simulink model "Dron_pid_XY"  (R2019a)
settings: Solver=FixedStepAuto  StartTime=0.0  StopTime=100  FixedStep=1e-5  RelTol=1e-3
values from neighbouring files (symbols this model uses):
  b = force_max_1 / omega_max ^ 2    (= 6.86183516529e-08)    [dron.m]
  d = 2e-9    (= 2e-09)    [dron.m]
  delay = 0.001    [dron.m]
  force_max = force_max_1 * 4    (= 47.088)    [dron.m]
  g = 9.81    [dron.m]
  Ixx = 0.02276    [dron.m]
  Iyy = Ixx    (= 0.02276)    [dron.m]
  Izz = 0.03132    [dron.m]
  k_x = 10    [dron.m]
  k_y = 10    [dron.m]
  k_z = 1    [dron.m]
  l = 0.225    [dron.m]
  m = 1    [dron.m]
  omega_max = 13098    [dron.m]
  torque_max_rp = omega_max ^ 2 * 2 * b * l    (= 5.2974)    [dron.m]
  torque_max_y = omega_max ^ 2 * 2 * d    (= 0.686230416)    [dron.m]
undefined symbols (not defined in the file or in its folder): sigbuilder_block
libraries: simulink_extras x9, simulink x6, powerlib_extras x1
settings Model: Creator=alber  LastModifiedBy=alber
settings DataIOCC: ReturnWorkspaceOutputs=off

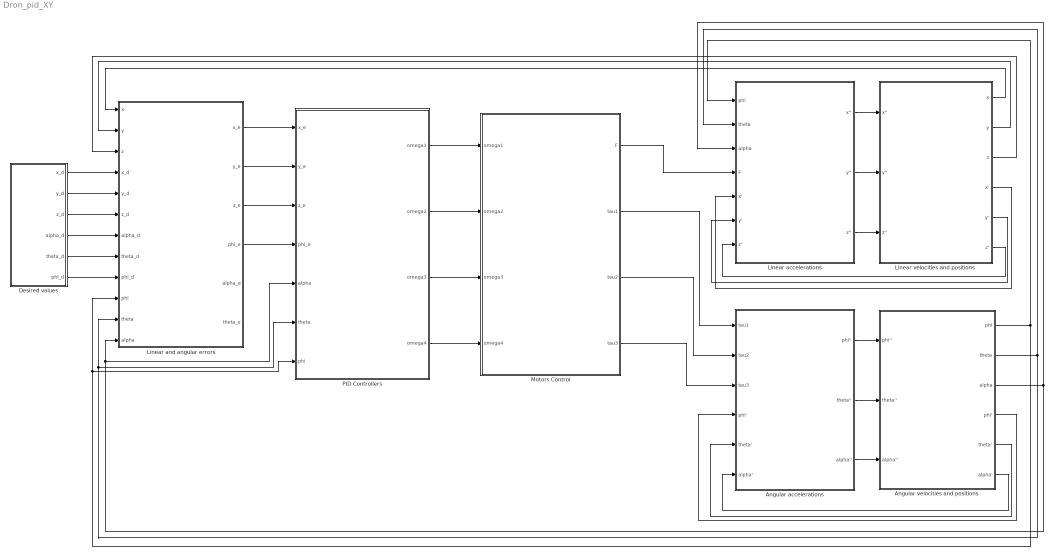
== system Dron_pid_XY ==
  Angular accelerations : Subsystem
  Angular velocities and positions : Subsystem
  Desired values : Subsystem
  Linear accelerations : Subsystem
  Linear and angular errors : Subsystem
  Linear velocities and positions : Subsystem
  Motors Control : Subsystem
  PID Controllers : Subsystem
  wires:
  Angular accelerations/1(phi'') -> Angular velocities and positions/1(phi'')
  Angular accelerations/2(theta'') -> Angular velocities and positions/2(theta'')
  Angular accelerations/3(alpha'') -> Angular velocities and positions/3(alpha'')
  Desired values/4(alpha_d) -> Linear and angular errors/7(alpha_d)
  Desired values/5(theta_d) -> Linear and angular errors/8(theta_d)
  Desired values/6(phi_d) -> Linear and angular errors/9(phi_d)
  Linear accelerations/3(z'') -> Linear velocities and positions/3(z'')
  Linear accelerations/2(y'') -> Linear velocities and positions/2(y'')
  Linear accelerations/1(x'') -> Linear velocities and positions/1(x'')
  Linear and angular errors/1(x_e) -> PID Controllers/1(x_e)
  Linear and angular errors/2(y_e) -> PID Controllers/2(y_e)
  Linear and angular errors/3(z_e) -> PID Controllers/3(z_e)
  Linear and angular errors/4(phi_e) -> PID Controllers/4(phi_e)
  PID Controllers/1(omega1) -> Motors Control/1(omega1)
  PID Controllers/2(omega2) -> Motors Control/2(omega2)
  PID Controllers/3(omega3) -> Motors Control/3(omega3)
  PID Controllers/4(omega4) -> Motors Control/4(omega4)
  Linear velocities and positions/6(z') -> Linear accelerations/7(z')
  Linear velocities and positions/5(y') -> Linear accelerations/6(y')
  Linear velocities and positions/4(x') -> Linear accelerations/5(x')
  Linear velocities and positions/1(x) -> Linear and angular errors/1(x)
  Linear velocities and positions/2(y) -> Linear and angular errors/2(y)
  Linear velocities and positions/3(z) -> Linear and angular errors/3(z)
  Angular velocities and positions/6(alpha') -> Angular accelerations/6(alpha')
  Angular velocities and positions/5(theta') -> Angular accelerations/5(theta')
  Angular velocities and positions/4(phi') -> Angular accelerations/4(phi')
  Motors Control/2(tau1) -> Angular accelerations/1(tau1)
  Motors Control/3(tau2) -> Angular accelerations/2(tau2)
  Motors Control/4(tau3) -> Angular accelerations/3(tau3)
  Motors Control/1(F) -> Linear accelerations/4(F)
  Angular velocities and positions/3(alpha) -> Linear accelerations/3(alpha), PID Controllers/5(alpha), Linear and angular errors/12(alpha)
  Angular velocities and positions/2(theta) -> Linear accelerations/2(theta), PID Controllers/6(theta), Linear and angular errors/11(theta)
  Angular velocities and positions/1(phi) -> Linear accelerations/1(phi), PID Controllers/7(phi), Linear and angular errors/10(phi)
  Desired values/1(x_d) -> Linear and angular errors/4(x_d)
  Desired values/2(y_d) -> Linear and angular errors/5(y_d)
  Desired values/3(z_d) -> Linear and angular errors/6(z_d)

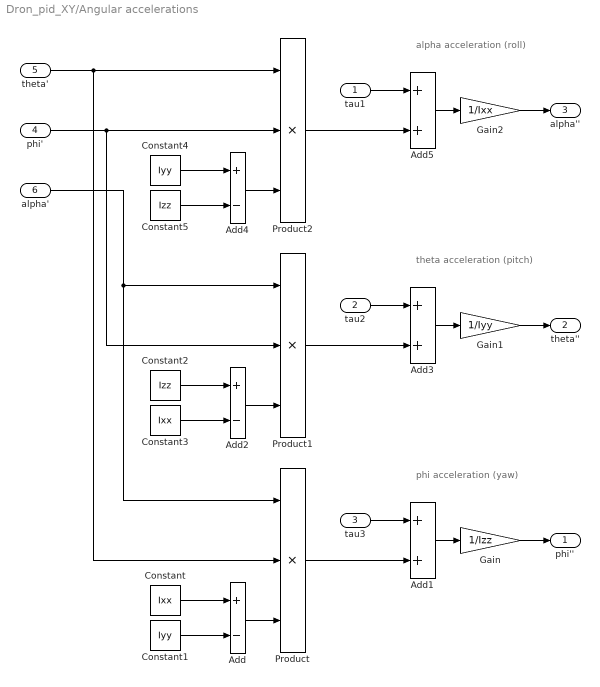
== system Dron_pid_XY/Angular accelerations ==
  note: alpha acceleration (roll)
  note: theta acceleration (pitch)
  note: phi acceleration (yaw)
  tau1 : Inport
  tau2 : Inport  Port=2
  tau3 : Inport  Port=3
  phi' : Inport  Port=4
  theta' : Inport  Port=5
  alpha' : Inport  Port=6
  Add : Sum  Inputs=+-
  Add1 : Sum
  Add2 : Sum  Inputs=+-
  Add3 : Sum
  Add4 : Sum  Inputs=+-
  Add5 : Sum
  Constant : Constant  Value=Ixx
  Constant1 : Constant  Value=Iyy
  Constant2 : Constant  Value=Izz
  Constant3 : Constant  Value=Ixx
  Constant4 : Constant  Value=Iyy
  Constant5 : Constant  Value=Izz
  Gain : Gain  Gain=1/Izz
  Gain1 : Gain  Gain=1/Iyy
  Gain2 : Gain  Gain=1/Ixx
  Product : Product  Inputs=3
  Product1 : Product  Inputs=3
  Product2 : Product  Inputs=3
  phi'' : Outport
  theta'' : Outport  Port=2
  alpha'' : Outport  Port=3
  wires:
  Constant2/1 -> Add2/1
  Add3/1 -> Gain1/1
  Constant1/1 -> Add/2
  Product2/1 -> Add5/2
  tau1/1 -> Add5/1
  Add1/1 -> Gain/1
  Add/1 -> Product/3
  Constant/1 -> Add/1
  Constant5/1 -> Add4/2
  Product1/1 -> Add3/2
  Add2/1 -> Product1/3
  tau2/1 -> Add3/1
  Constant3/1 -> Add2/2
  Add5/1 -> Gain2/1
  tau3/1 -> Add1/1
  Product/1 -> Add1/2
  Constant4/1 -> Add4/1
  Add4/1 -> Product2/3
  Gain2/1 -> alpha''/1
  Gain1/1 -> theta''/1
  Gain/1 -> phi''/1
  theta'/1 -> Product/2, Product2/1
  phi'/1 -> Product1/2, Product2/2
  alpha'/1 -> Product/1, Product1/1

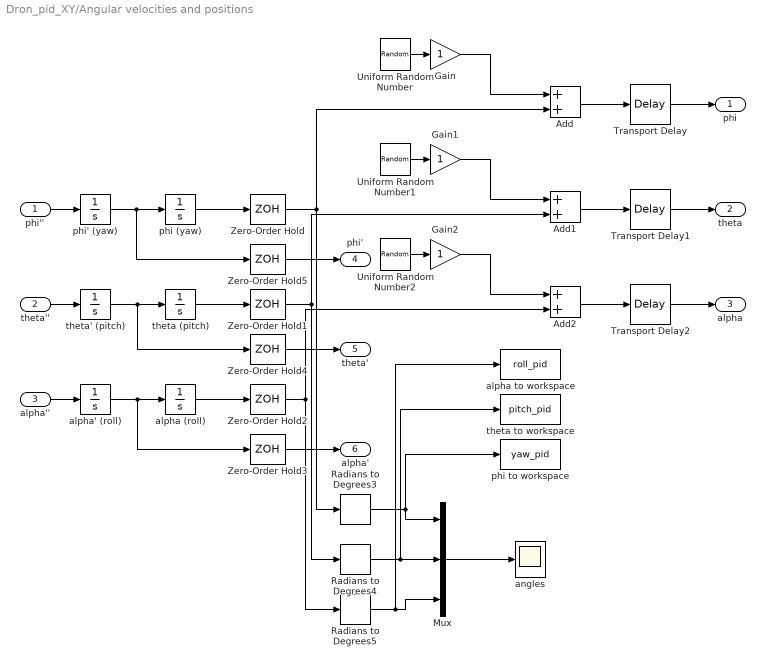
== system Dron_pid_XY/Angular velocities and positions ==
  phi'' : Inport
  theta'' : Inport  Port=2
  alpha'' : Inport  Port=3
  Add : Sum
  Add1 : Sum
  Add2 : Sum
  Gain : Gain
  Gain1 : Gain
  Gain2 : Gain
  Mux : Mux  Inputs=3
  Radians to Degrees3 : simulink_extras/Transformations/Radians to Degrees
  Radians to Degrees4 : simulink_extras/Transformations/Radians to Degrees
  Radians to Degrees5 : simulink_extras/Transformations/Radians to Degrees
  Transport Delay : TransportDelay  DelayTime=delay
  Transport Delay1 : TransportDelay  DelayTime=delay
  Transport Delay2 : TransportDelay  DelayTime=delay
  Uniform Random Number : UniformRandomNumber  Minimum=-0.005  Maximum=0.005  SampleTime=1e-4
  Uniform Random Number1 : UniformRandomNumber  Minimum=-0.005  Maximum=0.005  SampleTime=1e-4
  Uniform Random Number2 : UniformRandomNumber  Minimum=-0.005  Maximum=0.005  SampleTime=1e-4
  Zero-Order Hold{,1..5} (6 alike) : ZeroOrderHold  SampleTime=1e-4
  alpha (roll) : Integrator  LimitOutput=on  UpperSaturationLimit=pi  LowerSaturationLimit=-pi
  alpha to workspace : ToWorkspace  VariableName=roll_pid  SampleTime=1e-5
  alpha' (roll) : Integrator
  angles : Scope
  phi (yaw) : Integrator  LimitOutput=on  UpperSaturationLimit=pi  LowerSaturationLimit=-pi
  phi to workspace : ToWorkspace  VariableName=yaw_pid  SampleTime=1e-5
  phi' (yaw) : Integrator
  "theta (pitch) " : Integrator  LimitOutput=on  UpperSaturationLimit=pi  LowerSaturationLimit=-pi
  theta to workspace : ToWorkspace  VariableName=pitch_pid  SampleTime=1e-5
  theta' (pitch) : Integrator
  phi : Outport
  theta : Outport  Port=2
  alpha : Outport  Port=3
  phi' : Outport  Port=4
  theta' : Outport  Port=5
  alpha' : Outport  Port=6
  wires:
  phi (yaw)/1 -> Zero-Order Hold/1
  alpha' (roll)/1 -> Zero-Order Hold3/1, alpha (roll)/1
  theta' (pitch)/1 -> Zero-Order Hold4/1, "theta (pitch) "/1
  "theta (pitch) "/1 -> Zero-Order Hold1/1
  phi' (yaw)/1 -> Zero-Order Hold5/1, phi (yaw)/1
  theta''/1 -> theta' (pitch)/1
  alpha''/1 -> alpha' (roll)/1
  Zero-Order Hold1/1 -> Add1/2, Radians to Degrees4/1
  phi''/1 -> phi' (yaw)/1
  Zero-Order Hold/1 -> Radians to Degrees3/1, Add/2
  Zero-Order Hold2/1 -> Radians to Degrees5/1, Add2/2
  Radians to Degrees4/1 -> theta to workspace/1, Mux/2
  Radians to Degrees3/1 -> phi to workspace/1, Mux/1
  Radians to Degrees5/1 -> alpha to workspace/1, Mux/3
  Mux/1 -> angles/1
  alpha (roll)/1 -> Zero-Order Hold2/1
  Zero-Order Hold3/1 -> alpha'/1
  Zero-Order Hold4/1 -> theta'/1
  Zero-Order Hold5/1 -> phi'/1
  Uniform Random Number/1 -> Gain/1
  Uniform Random Number1/1 -> Gain1/1
  Uniform Random Number2/1 -> Gain2/1
  Add/1 -> Transport Delay/1
  Add1/1 -> Transport Delay1/1
  Add2/1 -> Transport Delay2/1
  Gain/1 -> Add/1
  Gain1/1 -> Add1/1
  Gain2/1 -> Add2/1
  Transport Delay/1 -> phi/1
  Transport Delay1/1 -> theta/1
  Transport Delay2/1 -> alpha/1

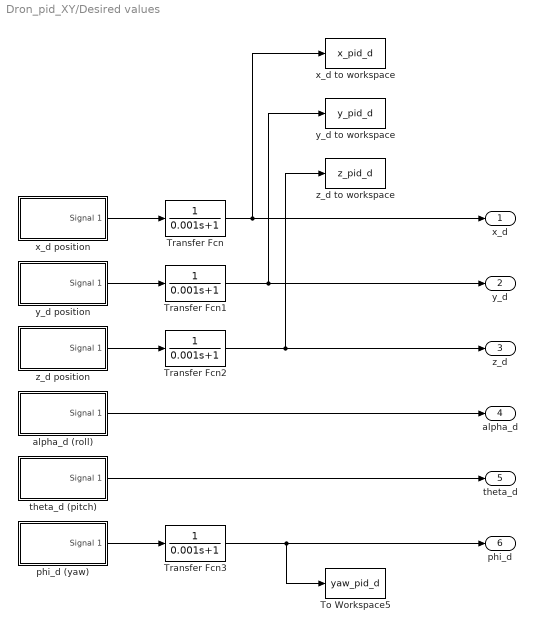
== system Dron_pid_XY/Desired values ==
  To Workspace5 : ToWorkspace  VariableName=yaw_pid_d  SampleTime=1e-5
  Transfer Fcn{,1..3} (4 alike) : TransferFcn  Denominator=[0.001 1]
  alpha_d (roll) : Subsystem  Tag=STV Subsys  LoadFcn=sigbuilder_block('load');  StartFcn=sigbuilder_block('start');  StopFcn=sigbuilder_block('stop');  ClipboardFcn=sigbuilder_block('clipboard');  mask(Sigbuilder block){tuvar=[0:10]}
      mask help: Simulink:masks:SigbuilderBlock_MD
      mask init:
      | if ~strcmp(get_param(bdroot(gcbh),'SimulationStatus'),'stopped') tuvar = sigbuilder_block('maskInit'); end
      settings: CopyFcn=sigbuilder_block('copy');  DeleteFcn=sigbuilder_block('delete');  ModelCloseFcn=sigbuilder_block('modelClose');  PreSaveFcn=sigbuilder_block('preSave');  PauseFcn=sigbuilder_block('pause');  ContinueFcn=sigbuilder_block('continue');  NameChangeFcn=sigbuilder_block('namechange');  OpenFcn=sigbuilder_block('open',[150.6 124.8 550.8 400.2 ]);  CloseFcn=sigbuilder_block('close');
      mask Display: plot(0, 0, 100, 100,[2, 2, 32, 32, 2], [68, 8, 8, 68, 68],[32, 2], [38, 38], [32, 19, 2],[53, 60, 44], [32, 17, 17, 2],[16, 16, 31, 31]);txt = getActiveGroup(gcbh);text(2, 100, txt,'verticalAlignment', 'top');
  phi_d (yaw) : Subsystem  Tag=STV Subsys  LoadFcn=sigbuilder_block('load');  StartFcn=sigbuilder_block('start');  StopFcn=sigbuilder_block('stop');  ClipboardFcn=sigbuilder_block('clipboard');  mask(Sigbuilder block){tuvar=[0:10]}
      mask help: Simulink:masks:SigbuilderBlock_MD
      mask init:
      | if ~strcmp(get_param(bdroot(gcbh),'SimulationStatus'),'stopped') tuvar = sigbuilder_block('maskInit'); end
      settings: CopyFcn=sigbuilder_block('copy');  DeleteFcn=sigbuilder_block('delete');  ModelCloseFcn=sigbuilder_block('modelClose');  PreSaveFcn=sigbuilder_block('preSave');  PauseFcn=sigbuilder_block('pause');  ContinueFcn=sigbuilder_block('continue');  NameChangeFcn=sigbuilder_block('namechange');  OpenFcn=sigbuilder_block('open',[595.8 77.4 550.8 361.2 ]);  CloseFcn=sigbuilder_block('close');
      mask Display: plot(0, 0, 100, 100,[2, 2, 32, 32, 2], [68, 8, 8, 68, 68],[32, 2], [38, 38], [32, 19, 2],[53, 60, 44], [32, 17, 17, 2],[16, 16, 31, 31]);txt = getActiveGroup(gcbh);text(2, 100, txt,'verticalAlignment', 'top');
  theta_d (pitch) : Subsystem  Tag=STV Subsys  LoadFcn=sigbuilder_block('load');  StartFcn=sigbuilder_block('start');  StopFcn=sigbuilder_block('stop');  ClipboardFcn=sigbuilder_block('clipboard');  mask(Sigbuilder block){tuvar=[0:10]}
      mask help: Simulink:masks:SigbuilderBlock_MD
      mask init:
      | if ~strcmp(get_param(bdroot(gcbh),'SimulationStatus'),'stopped') tuvar = sigbuilder_block('maskInit'); end
      settings: CopyFcn=sigbuilder_block('copy');  DeleteFcn=sigbuilder_block('delete');  ModelCloseFcn=sigbuilder_block('modelClose');  PreSaveFcn=sigbuilder_block('preSave');  PauseFcn=sigbuilder_block('pause');  ContinueFcn=sigbuilder_block('continue');  NameChangeFcn=sigbuilder_block('namechange');  OpenFcn=sigbuilder_block('open',[583.2 81.6 550.8 400.2 ]);  CloseFcn=sigbuilder_block('close');
      mask Display: plot(0, 0, 100, 100,[2, 2, 32, 32, 2], [68, 8, 8, 68, 68],[32, 2], [38, 38], [32, 19, 2],[53, 60, 44], [32, 17, 17, 2],[16, 16, 31, 31]);txt = getActiveGroup(gcbh);text(2, 100, txt,'verticalAlignment', 'top');
  x_d position : Subsystem  Tag=STV Subsys  LoadFcn=sigbuilder_block('load');  StartFcn=sigbuilder_block('start');  StopFcn=sigbuilder_block('stop');  ClipboardFcn=sigbuilder_block('clipboard');  mask(Sigbuilder block){tuvar=[0:10]}
      mask help: Simulink:masks:SigbuilderBlock_MD
      mask init:
      | if ~strcmp(get_param(bdroot(gcbh),'SimulationStatus'),'stopped') tuvar = sigbuilder_block('maskInit'); end
      settings: CopyFcn=sigbuilder_block('copy');  DeleteFcn=sigbuilder_block('delete');  ModelCloseFcn=sigbuilder_block('modelClose');  PreSaveFcn=sigbuilder_block('preSave');  PauseFcn=sigbuilder_block('pause');  ContinueFcn=sigbuilder_block('continue');  NameChangeFcn=sigbuilder_block('namechange');  OpenFcn=sigbuilder_block('open',[0.75 0.75 718.5 745.5 ]);  CloseFcn=sigbuilder_block('close');
      mask Display: plot(0, 0, 100, 100,[2, 2, 32, 32, 2], [68, 8, 8, 68, 68],[32, 2], [38, 38], [32, 19, 2],[53, 60, 44], [32, 17, 17, 2],[16, 16, 31, 31]);txt = getActiveGroup(gcbh);text(2, 100, txt,'verticalAlignment', 'top');
  x_d to workspace : ToWorkspace  VariableName=x_pid_d  SampleTime=1e-5
  y_d position : Subsystem  Tag=STV Subsys  LoadFcn=sigbuilder_block('load');  StartFcn=sigbuilder_block('start');  StopFcn=sigbuilder_block('stop');  ClipboardFcn=sigbuilder_block('clipboard');  mask(Sigbuilder block){tuvar=[0:10]}
      mask help: Simulink:masks:SigbuilderBlock_MD
      mask init:
      | if ~strcmp(get_param(bdroot(gcbh),'SimulationStatus'),'stopped') tuvar = sigbuilder_block('maskInit'); end
      settings: CopyFcn=sigbuilder_block('copy');  DeleteFcn=sigbuilder_block('delete');  ModelCloseFcn=sigbuilder_block('modelClose');  PreSaveFcn=sigbuilder_block('preSave');  PauseFcn=sigbuilder_block('pause');  ContinueFcn=sigbuilder_block('continue');  NameChangeFcn=sigbuilder_block('namechange');  OpenFcn=sigbuilder_block('open',[0.75 0.75 718.5 745.5 ]);  CloseFcn=sigbuilder_block('close');
      mask Display: plot(0, 0, 100, 100,[2, 2, 32, 32, 2], [68, 8, 8, 68, 68],[32, 2], [38, 38], [32, 19, 2],[53, 60, 44], [32, 17, 17, 2],[16, 16, 31, 31]);txt = getActiveGroup(gcbh);text(2, 100, txt,'verticalAlignment', 'top');
  y_d to workspace : ToWorkspace  VariableName=y_pid_d  SampleTime=1e-5
  z_d position : Subsystem  Tag=STV Subsys  LoadFcn=sigbuilder_block('load');  StartFcn=sigbuilder_block('start');  StopFcn=sigbuilder_block('stop');  ClipboardFcn=sigbuilder_block('clipboard');  mask(Sigbuilder block){tuvar=[0:10]}
      mask help: Simulink:masks:SigbuilderBlock_MD
      mask init:
      | if ~strcmp(get_param(bdroot(gcbh),'SimulationStatus'),'stopped') tuvar = sigbuilder_block('maskInit'); end
      settings: CopyFcn=sigbuilder_block('copy');  DeleteFcn=sigbuilder_block('delete');  ModelCloseFcn=sigbuilder_block('modelClose');  PreSaveFcn=sigbuilder_block('preSave');  PauseFcn=sigbuilder_block('pause');  ContinueFcn=sigbuilder_block('continue');  NameChangeFcn=sigbuilder_block('namechange');  OpenFcn=sigbuilder_block('open',[112.5 10.5 574.5 585.75 ]);  CloseFcn=sigbuilder_block('close');
      mask Display: plot(0, 0, 100, 100,[2, 2, 32, 32, 2], [68, 8, 8, 68, 68],[32, 2], [38, 38], [32, 19, 2],[53, 60, 44], [32, 17, 17, 2],[16, 16, 31, 31]);txt = getActiveGroup(gcbh);text(2, 100, txt,'verticalAlignment', 'top');
  z_d to workspace : ToWorkspace  VariableName=z_pid_d  SampleTime=1e-5
  x_d : Outport
  y_d : Outport  Port=2
  z_d : Outport  Port=3
  alpha_d : Outport  Port=4
  theta_d : Outport  Port=5
  phi_d : Outport  Port=6
  wires:
  alpha_d (roll)/1(Signal 1) -> alpha_d/1
  phi_d (yaw)/1(Signal 1) -> Transfer Fcn3/1
  theta_d (pitch)/1(Signal 1) -> theta_d/1
  z_d position/1(Signal 1) -> Transfer Fcn2/1
  y_d position/1(Signal 1) -> Transfer Fcn1/1
  x_d position/1(Signal 1) -> Transfer Fcn/1
  Transfer Fcn/1 -> x_d/1, x_d to workspace/1
  Transfer Fcn1/1 -> y_d/1, y_d to workspace/1
  Transfer Fcn2/1 -> z_d/1, z_d to workspace/1
  Transfer Fcn3/1 -> phi_d/1, To Workspace5/1

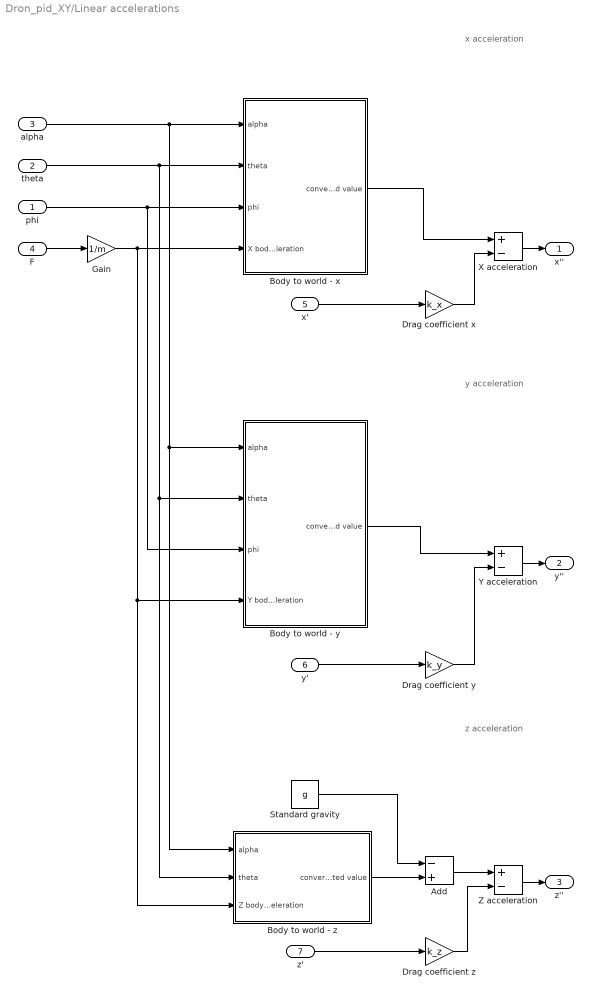
== system Dron_pid_XY/Linear accelerations ==
  note: z acceleration
  note: y acceleration
  note: x acceleration
  phi : Inport
  theta : Inport  Port=2
  alpha : Inport  Port=3
  F : Inport  Port=4
  x' : Inport  Port=5
  y' : Inport  Port=6
  z' : Inport  Port=7
  Add : Sum  Inputs=-+
  Body to world - x : Subsystem
  Body to world - y : Subsystem
  Body to world - z : Subsystem
  Drag coefficient x : Gain  Gain=k_x
  Drag coefficient y : Gain  Gain=k_y
  Drag coefficient z : Gain  Gain=k_z
  Gain : Gain  Gain=1/m
  Standard gravity : Constant  Value=g
  X acceleration : Sum  Inputs=+-
  Y acceleration : Sum  Inputs=+-
  Z acceleration : Sum  Inputs=+-
  x'' : Outport
  y'' : Outport  Port=2
  z'' : Outport  Port=3
  wires:
  theta/1 -> Body to world - z/2(theta), Body to world - y/2(theta), Body to world - x/2(theta)
  alpha/1 -> Body to world - z/1(alpha), Body to world - y/1(alpha), Body to world - x/1(alpha)
  phi/1 -> Body to world - y/3(phi), Body to world - x/3("phi ")
  Body to world - z/1(converted value) -> Add/2
  Standard gravity/1 -> Add/1
  F/1 -> Gain/1
  Add/1 -> Z acceleration/1
  Z acceleration/1 -> z''/1
  Y acceleration/1 -> y''/1
  X acceleration/1 -> x''/1
  Drag coefficient z/1 -> Z acceleration/2
  Drag coefficient y/1 -> Y acceleration/2
  Drag coefficient x/1 -> X acceleration/2
  Gain/1 -> Body to world - z/3(Z body acceleration), Body to world - y/4(Y body acceleration), Body to world - x/4(X body acceleration)
  Body to world - x/1(converted value) -> X acceleration/1
  Body to world - y/1(converted value) -> Y acceleration/1
  x'/1 -> Drag coefficient x/1
  y'/1 -> Drag coefficient y/1
  z'/1 -> Drag coefficient z/1

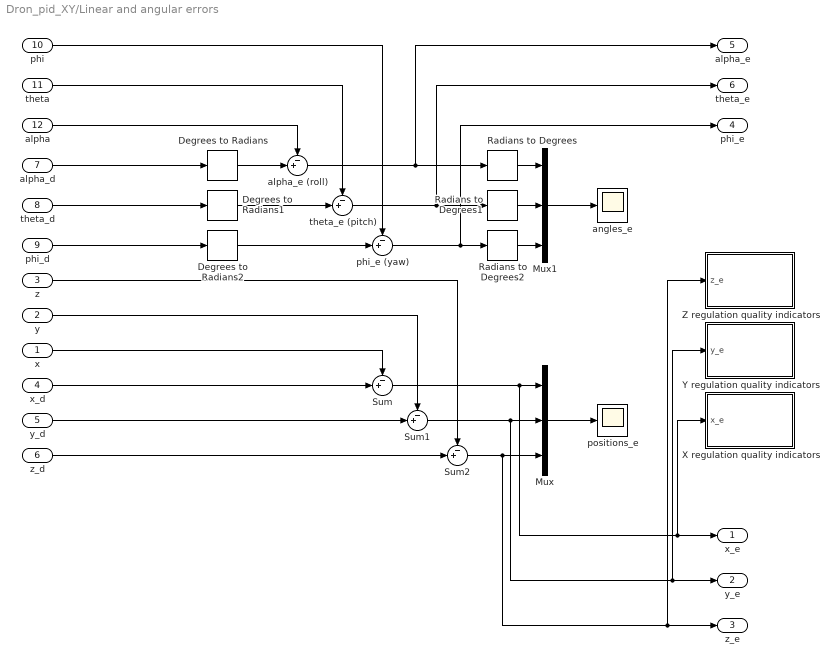
== system Dron_pid_XY/Linear and angular errors ==
  x : Inport
  y : Inport  Port=2
  z : Inport  Port=3
  x_d : Inport  Port=4
  y_d : Inport  Port=5
  z_d : Inport  Port=6
  alpha_d : Inport  Port=7
  theta_d : Inport  Port=8
  phi_d : Inport  Port=9
  phi : Inport  Port=10
  theta : Inport  Port=11
  alpha : Inport  Port=12
  Degrees to Radians : simulink_extras/Transformations/Degrees to Radians
  Degrees to Radians1 : simulink_extras/Transformations/Degrees to Radians
  Degrees to Radians2 : simulink_extras/Transformations/Degrees to Radians
  Mux : Mux  Inputs=3
  Mux1 : Mux  Inputs=3
  Radians to Degrees : simulink_extras/Transformations/Radians to Degrees
  Radians to Degrees1 : simulink_extras/Transformations/Radians to Degrees
  Radians to Degrees2 : simulink_extras/Transformations/Radians to Degrees
  Sum : Sum  Inputs=-+|
  Sum1 : Sum  Inputs=-+|
  Sum2 : Sum  Inputs=-+|
  X regulation quality indicators : Subsystem
  Y regulation quality indicators : Subsystem
  Z regulation quality indicators : Subsystem
  alpha_e (roll) : Sum  Inputs=-+|
  angles_e : Scope
  phi_e (yaw) : Sum  Inputs=-+|
  positions_e : Scope
  theta_e (pitch) : Sum  Inputs=-+|
  x_e : Outport
  y_e : Outport  Port=2
  z_e : Outport  Port=3
  phi_e : Outport  Port=4
  alpha_e : Outport  Port=5
  theta_e : Outport  Port=6
  wires:
  Mux1/1 -> angles_e/1
  Radians to Degrees/1 -> Mux1/1
  Radians to Degrees1/1 -> Mux1/2
  Radians to Degrees2/1 -> Mux1/3
  Sum/1 -> X regulation quality indicators/1(x_e), x_e/1, Mux/1
  Sum1/1 -> Y regulation quality indicators/1(y_e), y_e/1, Mux/2
  alpha_e (roll)/1 -> alpha_e/1, Radians to Degrees/1
  theta_e (pitch)/1 -> theta_e/1, Radians to Degrees1/1
  phi_e (yaw)/1 -> phi_e/1, Radians to Degrees2/1
  alpha_d/1 -> Degrees to Radians/1
  theta_d/1 -> Degrees to Radians1/1
  phi_d/1 -> Degrees to Radians2/1
  z_d/1 -> Sum2/2
  y_d/1 -> Sum1/2
  alpha/1 -> alpha_e (roll)/1
  theta/1 -> theta_e (pitch)/1
  phi/1 -> phi_e (yaw)/1
  x/1 -> Sum/1
  y/1 -> Sum1/1
  z/1 -> Sum2/1
  Mux/1 -> positions_e/1
  Degrees to Radians/1 -> alpha_e (roll)/2
  Degrees to Radians1/1 -> theta_e (pitch)/2
  Degrees to Radians2/1 -> phi_e (yaw)/2
  x_d/1 -> Sum/2
  Sum2/1 -> Z regulation quality indicators/1(z_e), z_e/1, Mux/3

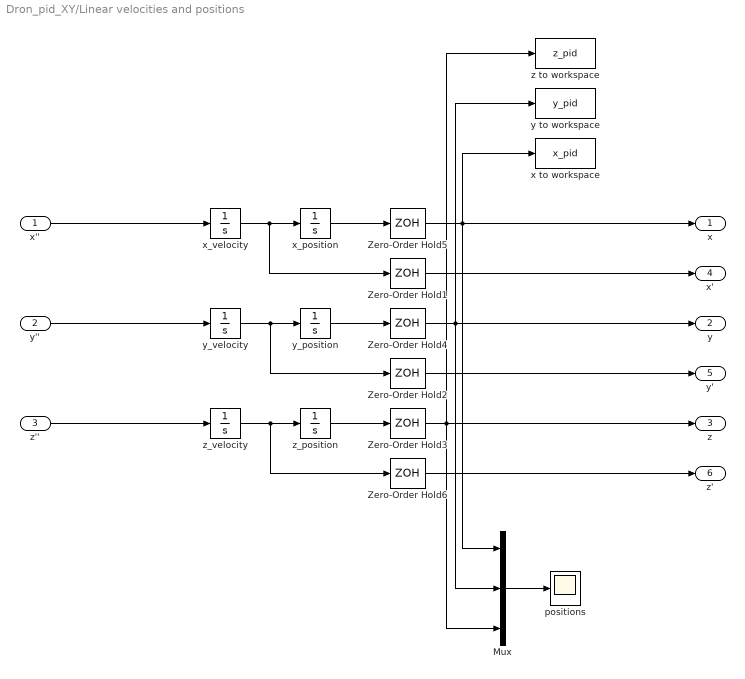
== system Dron_pid_XY/Linear velocities and positions ==
  x'' : Inport
  y'' : Inport  Port=2
  z'' : Inport  Port=3
  Mux : Mux  Inputs=3
  Zero-Order Hold{1..6} (6 alike) : ZeroOrderHold  SampleTime=1e-4
  positions : Scope
  x to workspace : ToWorkspace  VariableName=x_pid  SampleTime=1e-5
  x_position : Integrator
  x_velocity : Integrator
  y to workspace : ToWorkspace  VariableName=y_pid  SampleTime=1e-5
  y_position : Integrator
  y_velocity : Integrator
  z to workspace : ToWorkspace  VariableName=z_pid  SampleTime=1e-5
  z_position : Integrator  LimitOutput=on  LowerSaturationLimit=0
  z_velocity : Integrator
  x : Outport
  y : Outport  Port=2
  z : Outport  Port=3
  x' : Outport  Port=4
  y' : Outport  Port=5
  z' : Outport  Port=6
  wires:
  x_velocity/1 -> Zero-Order Hold1/1, x_position/1
  z_position/1 -> Zero-Order Hold3/1
  Zero-Order Hold4/1 -> Mux/2, y to workspace/1, y/1
  Zero-Order Hold5/1 -> x to workspace/1, Mux/1, x/1
  y_position/1 -> Zero-Order Hold4/1
  z_velocity/1 -> Zero-Order Hold6/1, z_position/1
  y_velocity/1 -> Zero-Order Hold2/1, y_position/1
  x_position/1 -> Zero-Order Hold5/1
  x''/1 -> x_velocity/1
  z''/1 -> z_velocity/1
  y''/1 -> y_velocity/1
  Zero-Order Hold3/1 -> Mux/3, z to workspace/1, z/1
  Mux/1 -> positions/1
  Zero-Order Hold1/1 -> x'/1
  Zero-Order Hold2/1 -> y'/1
  Zero-Order Hold6/1 -> z'/1

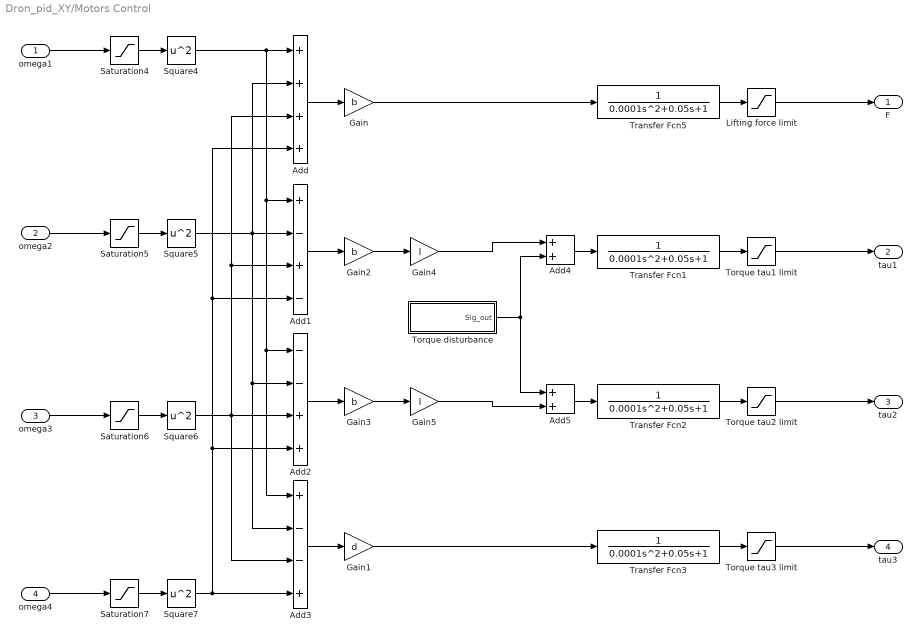
== system Dron_pid_XY/Motors Control ==
  omega1 : Inport
  omega2 : Inport  Port=2
  omega3 : Inport  Port=3
  omega4 : Inport  Port=4
  Add : Sum  Inputs=4
  Add1 : Sum  Inputs=+-+-
  Add2 : Sum  Inputs=--++
  Add3 : Sum  Inputs=+--+
  Add4 : Sum
  Add5 : Sum
  Gain : Gain  Gain=b
  Gain1 : Gain  Gain=d
  Gain2 : Gain  Gain=b
  Gain3 : Gain  Gain=b
  Gain4 : Gain  Gain=l
  Gain5 : Gain  Gain=l
  Lifting force limit : Saturate  UpperLimit=force_max  LowerLimit=0
  Saturation{4..7} (4 alike) : Saturate  UpperLimit=omega_max  LowerLimit=0
  Square{4..7} (4 alike) : Math  Operator=square  SaturateOnIntegerOverflow=on
  Torque disturbance : Subsystem
  Torque tau1 limit : Saturate  UpperLimit=torque_max_rp  LowerLimit=-torque_max_rp
  Torque tau2 limit : Saturate  UpperLimit=torque_max_rp  LowerLimit=-torque_max_rp
  Torque tau3 limit : Saturate  UpperLimit=torque_max_y  LowerLimit=-torque_max_y
  Transfer Fcn{1..3,5} (4 alike) : TransferFcn  Denominator=[0.0001 0.05 1]
  F : Outport
  tau1 : Outport  Port=2
  tau2 : Outport  Port=3
  tau3 : Outport  Port=4
  wires:
  omega3/1 -> Saturation6/1
  omega1/1 -> Saturation4/1
  omega4/1 -> Saturation7/1
  omega2/1 -> Saturation5/1
  Add2/1 -> Gain3/1
  Add1/1 -> Gain2/1
  Add/1 -> Gain/1
  Add3/1 -> Gain1/1
  Saturation4/1 -> Square4/1
  Saturation5/1 -> Square5/1
  Saturation6/1 -> Square6/1
  Saturation7/1 -> Square7/1
  Lifting force limit/1 -> F/1
  Torque tau3 limit/1 -> tau3/1
  Square4/1 -> Add3/1, Add2/1, Add1/1, Add/1
  Square5/1 -> Add/2, Add3/2, Add2/2, Add1/2
  Square6/1 -> Add/3, Add1/3, Add2/3, Add3/3
  Square7/1 -> Add/4, Add1/4, Add2/4, Add3/4
  Gain2/1 -> Gain4/1
  Gain3/1 -> Gain5/1
  Torque tau1 limit/1 -> tau1/1
  Torque tau2 limit/1 -> tau2/1
  Gain/1 -> Transfer Fcn5/1
  Add4/1 -> Transfer Fcn1/1
  Add5/1 -> Transfer Fcn2/1
  Gain1/1 -> Transfer Fcn3/1
  Gain5/1 -> Add5/2
  Gain4/1 -> Add4/1
  Torque disturbance/1(Sig_out) -> Add5/1, Add4/2
  Transfer Fcn5/1 -> Lifting force limit/1
  Transfer Fcn1/1 -> Torque tau1 limit/1
  Transfer Fcn2/1 -> Torque tau2 limit/1
  Transfer Fcn3/1 -> Torque tau3 limit/1

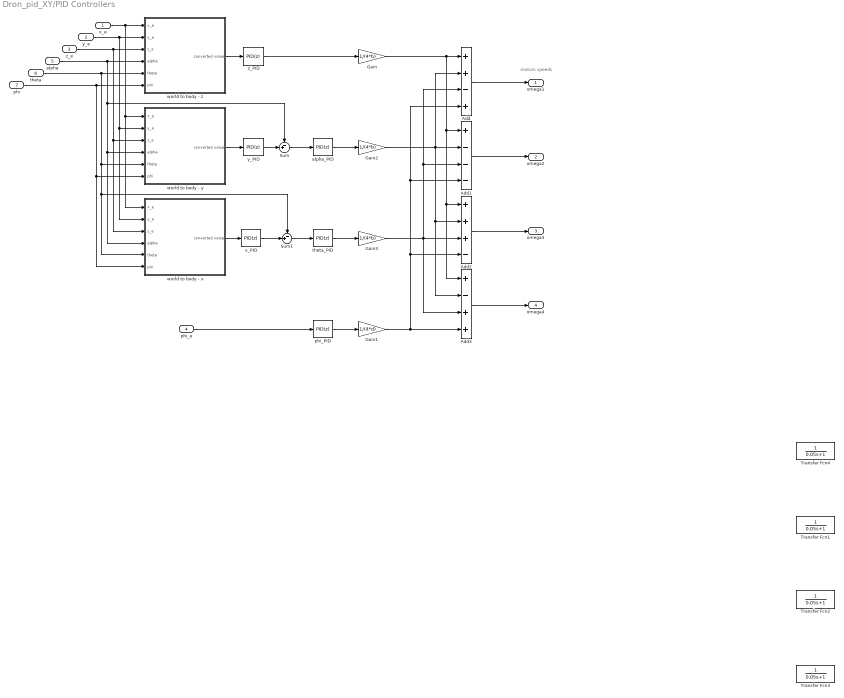
== system Dron_pid_XY/PID Controllers ==
  note: motors speeds
  x_e : Inport
  y_e : Inport  Port=2
  z_e : Inport  Port=3
  phi_e : Inport  Port=4
  alpha : Inport  Port=5
  theta : Inport  Port=6
  phi : Inport  Port=7
  Add : Sum  Inputs=++-+
  Add1 : Sum  Inputs=+---
  Add2 : Sum  Inputs=+++-
  Add3 : Sum  Inputs=+-++
  Gain : Gain  Gain=1/(4*b)
  Gain1 : Gain  Gain=1/(4*d)
  Gain2 : Gain  Gain=1/(4*b)
  Gain3 : Gain  Gain=1/(4*b)
  Sum : Sum  Inputs=-+|
  Sum1 : Sum  Inputs=-+|
  Transfer Fcn{1..4} (4 alike) : TransferFcn  Denominator=[0.05 1]
  alpha_PID : simulink/Continuous/PID Controller  Controller=PID  Form=Parallel  TimeDomain=Discrete-time  SampleTime=5e-4  IntegratorMethod=Forward Euler  FilterMethod=Forward Euler  ControllerParametersSource=internal  P=0.0003  I=0.00015  D=0.0001  UseFilter=on  N=100  TunerSelectOption=Transfer Function Based (PID Tuner App)  InitialConditionSource=internal  InitialConditionForIntegrator=0  InitialConditionForFilter=0  DifferentiatorICPrevScaledInput=0  ExternalReset=none  TrackingMode=off  Kt=1  LimitOutput=off  UpperSaturationLimit=inf  LowerSaturationLimit=-inf  LinearizeAsGain=on  AntiWindupMode=none  Kb=1  POutMin=[]  POutMax=[]  IOutMin=[]  IOutMax=[]  DOutMin=[]  DOutMax=[]  NOutMin=[]  NOutMax=[]  SumOutMin=[]  SumOutMax=[]  SaturationOutMin=[]  SaturationOutMax=[]  PParamMin=[]  PParamMax=[]  IParamMin=[]  IParamMax=[]  DParamMin=[]  DParamMax=[]  NParamMin=[]  NParamMax=[]  KbParamMin=[]  KbParamMax=[]  KtParamMin=[]  KtParamMax=[]  KbOutMin=[]  KbOutMax=[]  KtOutMin=[]  KtOutMax=[]  IntegratorOutMin=[]  IntegratorOutMax=[]  FilterOutMin=[]  FilterOutMax=[]  SumI1OutMin=[]  SumI1OutMax=[]  SumI2OutMin=[]  SumI2OutMax=[]  SumI3OutMin=[]  SumI3OutMax=[]  SumI4OutMin=[]  SumI4OutMax=[]  SumDOutMin=[]  SumDOutMax=[]  DifferentiatorOutMin=[]  DifferentiatorOutMax=[]  FilterDiffOutCoefMin=[]  FilterDiffOutCoefMax=[]  ReciprocalOutMin=[]  ReciprocalOutMax=[]  SumDenOutMin=[]  SumDenOutMax=[]  SumNumOutMin=[]  SumNumOutMax=[]  DivideOutMin=[]  DivideOutMax=[]  IntegratorContinuousStateAttributes=''  IntegratorStateMustResolveToSignalObject=off  IntegratorRTWStateStorageClass=Auto  FilterContinuousStateAttributes=''  FilterStateMustResolveToSignalObject=off  FilterRTWStateStorageClass=Auto  ParallelPVariant=InternalParameters  IdealPVariant=Disabled  IVariant=InternalParameters  DVariant=InternalParameters  IntegratorVariant=Discrete  SatVariant=Disabled  AWVariant=Passthrough  PCopyVariant=Disabled  TRVariant=Disabled  FdbkBlocksVariant=Forward  IdealPFdbkVariant=Disabled  SatFdbkVariant=Disabled  DerivativeFilterVariant=ForwardEulerFilter  NVariant=InternalParameters  NCopyVariant=Disabled  FilterICVariant=InternalICsFilter  IntegratorICVariant=InternalICs  ExternalResetVariant=Disabled  TRSumVariant=Passthrough  SumFdbkVariant=Disabled  SumVariant=Sum_PID
  phi_PID : simulink/Continuous/PID Controller  Controller=PID  Form=Parallel  TimeDomain=Discrete-time  SampleTime=5e-4  IntegratorMethod=Forward Euler  FilterMethod=Forward Euler  ControllerParametersSource=internal  P=0.0001  I=0.0001  D=0.0001  UseFilter=on  N=100  TunerSelectOption=Transfer Function Based (PID Tuner App)  InitialConditionSource=internal  InitialConditionForIntegrator=0  InitialConditionForFilter=0  DifferentiatorICPrevScaledInput=0  ExternalReset=none  TrackingMode=off  Kt=1  LimitOutput=off  UpperSaturationLimit=inf  LowerSaturationLimit=-inf  LinearizeAsGain=on  AntiWindupMode=none  Kb=1  POutMin=[]  POutMax=[]  IOutMin=[]  IOutMax=[]  DOutMin=[]  DOutMax=[]  NOutMin=[]  NOutMax=[]  SumOutMin=[]  SumOutMax=[]  SaturationOutMin=[]  SaturationOutMax=[]  PParamMin=[]  PParamMax=[]  IParamMin=[]  IParamMax=[]  DParamMin=[]  DParamMax=[]  NParamMin=[]  NParamMax=[]  KbParamMin=[]  KbParamMax=[]  KtParamMin=[]  KtParamMax=[]  KbOutMin=[]  KbOutMax=[]  KtOutMin=[]  KtOutMax=[]  IntegratorOutMin=[]  IntegratorOutMax=[]  FilterOutMin=[]  FilterOutMax=[]  SumI1OutMin=[]  SumI1OutMax=[]  SumI2OutMin=[]  SumI2OutMax=[]  SumI3OutMin=[]  SumI3OutMax=[]  SumI4OutMin=[]  SumI4OutMax=[]  SumDOutMin=[]  SumDOutMax=[]  DifferentiatorOutMin=[]  DifferentiatorOutMax=[]  FilterDiffOutCoefMin=[]  FilterDiffOutCoefMax=[]  ReciprocalOutMin=[]  ReciprocalOutMax=[]  SumDenOutMin=[]  SumDenOutMax=[]  SumNumOutMin=[]  SumNumOutMax=[]  DivideOutMin=[]  DivideOutMax=[]  IntegratorContinuousStateAttributes=''  IntegratorStateMustResolveToSignalObject=off  IntegratorRTWStateStorageClass=Auto  FilterContinuousStateAttributes=''  FilterStateMustResolveToSignalObject=off  FilterRTWStateStorageClass=Auto  ParallelPVariant=InternalParameters  IdealPVariant=Disabled  IVariant=InternalParameters  DVariant=InternalParameters  IntegratorVariant=Discrete  SatVariant=Disabled  AWVariant=Passthrough  PCopyVariant=Disabled  TRVariant=Disabled  FdbkBlocksVariant=Forward  IdealPFdbkVariant=Disabled  SatFdbkVariant=Disabled  DerivativeFilterVariant=ForwardEulerFilter  NVariant=InternalParameters  NCopyVariant=Disabled  FilterICVariant=InternalICsFilter  IntegratorICVariant=InternalICs  ExternalResetVariant=Disabled  TRSumVariant=Passthrough  SumFdbkVariant=Disabled  SumVariant=Sum_PID
  theta_PID : simulink/Continuous/PID Controller  Controller=PID  Form=Parallel  TimeDomain=Discrete-time  SampleTime=5e-4  IntegratorMethod=Forward Euler  FilterMethod=Forward Euler  ControllerParametersSource=internal  P=0.0003  I=0.00015  D=0.0001  UseFilter=on  N=100  TunerSelectOption=Transfer Function Based (PID Tuner App)  InitialConditionSource=internal  InitialConditionForIntegrator=0  InitialConditionForFilter=0  DifferentiatorICPrevScaledInput=0  ExternalReset=none  TrackingMode=off  Kt=1  LimitOutput=off  UpperSaturationLimit=inf  LowerSaturationLimit=-inf  LinearizeAsGain=on  AntiWindupMode=none  Kb=1  POutMin=[]  POutMax=[]  IOutMin=[]  IOutMax=[]  DOutMin=[]  DOutMax=[]  NOutMin=[]  NOutMax=[]  SumOutMin=[]  SumOutMax=[]  SaturationOutMin=[]  SaturationOutMax=[]  PParamMin=[]  PParamMax=[]  IParamMin=[]  IParamMax=[]  DParamMin=[]  DParamMax=[]  NParamMin=[]  NParamMax=[]  KbParamMin=[]  KbParamMax=[]  KtParamMin=[]  KtParamMax=[]  KbOutMin=[]  KbOutMax=[]  KtOutMin=[]  KtOutMax=[]  IntegratorOutMin=[]  IntegratorOutMax=[]  FilterOutMin=[]  FilterOutMax=[]  SumI1OutMin=[]  SumI1OutMax=[]  SumI2OutMin=[]  SumI2OutMax=[]  SumI3OutMin=[]  SumI3OutMax=[]  SumI4OutMin=[]  SumI4OutMax=[]  SumDOutMin=[]  SumDOutMax=[]  DifferentiatorOutMin=[]  DifferentiatorOutMax=[]  FilterDiffOutCoefMin=[]  FilterDiffOutCoefMax=[]  ReciprocalOutMin=[]  ReciprocalOutMax=[]  SumDenOutMin=[]  SumDenOutMax=[]  SumNumOutMin=[]  SumNumOutMax=[]  DivideOutMin=[]  DivideOutMax=[]  IntegratorContinuousStateAttributes=''  IntegratorStateMustResolveToSignalObject=off  IntegratorRTWStateStorageClass=Auto  FilterContinuousStateAttributes=''  FilterStateMustResolveToSignalObject=off  FilterRTWStateStorageClass=Auto  ParallelPVariant=InternalParameters  IdealPVariant=Disabled  IVariant=InternalParameters  DVariant=InternalParameters  IntegratorVariant=Discrete  SatVariant=Disabled  AWVariant=Passthrough  PCopyVariant=Disabled  TRVariant=Disabled  FdbkBlocksVariant=Forward  IdealPFdbkVariant=Disabled  SatFdbkVariant=Disabled  DerivativeFilterVariant=ForwardEulerFilter  NVariant=InternalParameters  NCopyVariant=Disabled  FilterICVariant=InternalICsFilter  IntegratorICVariant=InternalICs  ExternalResetVariant=Disabled  TRSumVariant=Passthrough  SumFdbkVariant=Disabled  SumVariant=Sum_PID
  world to body - x : Subsystem
  world to body - y : Subsystem
  world to body - z : Subsystem
  x_PID : simulink/Continuous/PID Controller  Controller=PID  Form=Parallel  TimeDomain=Discrete-time  SampleTime=1e-3  IntegratorMethod=Forward Euler  FilterMethod=Forward Euler  ControllerParametersSource=internal  P=2  I=0.5  D=0  UseFilter=on  N=100  TunerSelectOption=Transfer Function Based (PID Tuner App)  InitialConditionSource=internal  InitialConditionForIntegrator=0  InitialConditionForFilter=0  DifferentiatorICPrevScaledInput=0  ExternalReset=none  TrackingMode=off  Kt=1  LimitOutput=off  UpperSaturationLimit=inf  LowerSaturationLimit=-inf  LinearizeAsGain=on  AntiWindupMode=none  Kb=1  POutMin=[]  POutMax=[]  IOutMin=[]  IOutMax=[]  DOutMin=[]  DOutMax=[]  NOutMin=[]  NOutMax=[]  SumOutMin=[]  SumOutMax=[]  SaturationOutMin=[]  SaturationOutMax=[]  PParamMin=[]  PParamMax=[]  IParamMin=[]  IParamMax=[]  DParamMin=[]  DParamMax=[]  NParamMin=[]  NParamMax=[]  KbParamMin=[]  KbParamMax=[]  KtParamMin=[]  KtParamMax=[]  KbOutMin=[]  KbOutMax=[]  KtOutMin=[]  KtOutMax=[]  IntegratorOutMin=[]  IntegratorOutMax=[]  FilterOutMin=[]  FilterOutMax=[]  SumI1OutMin=[]  SumI1OutMax=[]  SumI2OutMin=[]  SumI2OutMax=[]  SumI3OutMin=[]  SumI3OutMax=[]  SumI4OutMin=[]  SumI4OutMax=[]  SumDOutMin=[]  SumDOutMax=[]  DifferentiatorOutMin=[]  DifferentiatorOutMax=[]  FilterDiffOutCoefMin=[]  FilterDiffOutCoefMax=[]  ReciprocalOutMin=[]  ReciprocalOutMax=[]  SumDenOutMin=[]  SumDenOutMax=[]  SumNumOutMin=[]  SumNumOutMax=[]  DivideOutMin=[]  DivideOutMax=[]  IntegratorContinuousStateAttributes=''  IntegratorStateMustResolveToSignalObject=off  IntegratorRTWStateStorageClass=Auto  FilterContinuousStateAttributes=''  FilterStateMustResolveToSignalObject=off  FilterRTWStateStorageClass=Auto  ParallelPVariant=InternalParameters  IdealPVariant=Disabled  IVariant=InternalParameters  DVariant=InternalParameters  IntegratorVariant=Discrete  SatVariant=Disabled  AWVariant=Passthrough  PCopyVariant=Disabled  TRVariant=Disabled  FdbkBlocksVariant=Forward  IdealPFdbkVariant=Disabled  SatFdbkVariant=Disabled  DerivativeFilterVariant=ForwardEulerFilter  NVariant=InternalParameters  NCopyVariant=Disabled  FilterICVariant=InternalICsFilter  IntegratorICVariant=InternalICs  ExternalResetVariant=Disabled  TRSumVariant=Passthrough  SumFdbkVariant=Disabled  SumVariant=Sum_PID
  y_PID : simulink/Continuous/PID Controller  Controller=PID  Form=Parallel  TimeDomain=Discrete-time  SampleTime=1e-3  IntegratorMethod=Forward Euler  FilterMethod=Forward Euler  ControllerParametersSource=internal  P=2  I=0.5  D=0  UseFilter=on  N=100  TunerSelectOption=Transfer Function Based (PID Tuner App)  InitialConditionSource=internal  InitialConditionForIntegrator=0  InitialConditionForFilter=0  DifferentiatorICPrevScaledInput=0  ExternalReset=none  TrackingMode=off  Kt=1  LimitOutput=off  UpperSaturationLimit=inf  LowerSaturationLimit=-inf  LinearizeAsGain=on  AntiWindupMode=none  Kb=1  POutMin=[]  POutMax=[]  IOutMin=[]  IOutMax=[]  DOutMin=[]  DOutMax=[]  NOutMin=[]  NOutMax=[]  SumOutMin=[]  SumOutMax=[]  SaturationOutMin=[]  SaturationOutMax=[]  PParamMin=[]  PParamMax=[]  IParamMin=[]  IParamMax=[]  DParamMin=[]  DParamMax=[]  NParamMin=[]  NParamMax=[]  KbParamMin=[]  KbParamMax=[]  KtParamMin=[]  KtParamMax=[]  KbOutMin=[]  KbOutMax=[]  KtOutMin=[]  KtOutMax=[]  IntegratorOutMin=[]  IntegratorOutMax=[]  FilterOutMin=[]  FilterOutMax=[]  SumI1OutMin=[]  SumI1OutMax=[]  SumI2OutMin=[]  SumI2OutMax=[]  SumI3OutMin=[]  SumI3OutMax=[]  SumI4OutMin=[]  SumI4OutMax=[]  SumDOutMin=[]  SumDOutMax=[]  DifferentiatorOutMin=[]  DifferentiatorOutMax=[]  FilterDiffOutCoefMin=[]  FilterDiffOutCoefMax=[]  ReciprocalOutMin=[]  ReciprocalOutMax=[]  SumDenOutMin=[]  SumDenOutMax=[]  SumNumOutMin=[]  SumNumOutMax=[]  DivideOutMin=[]  DivideOutMax=[]  IntegratorContinuousStateAttributes=''  IntegratorStateMustResolveToSignalObject=off  IntegratorRTWStateStorageClass=Auto  FilterContinuousStateAttributes=''  FilterStateMustResolveToSignalObject=off  FilterRTWStateStorageClass=Auto  ParallelPVariant=InternalParameters  IdealPVariant=Disabled  IVariant=InternalParameters  DVariant=InternalParameters  IntegratorVariant=Discrete  SatVariant=Disabled  AWVariant=Passthrough  PCopyVariant=Disabled  TRVariant=Disabled  FdbkBlocksVariant=Forward  IdealPFdbkVariant=Disabled  SatFdbkVariant=Disabled  DerivativeFilterVariant=ForwardEulerFilter  NVariant=InternalParameters  NCopyVariant=Disabled  FilterICVariant=InternalICsFilter  IntegratorICVariant=InternalICs  ExternalResetVariant=Disabled  TRSumVariant=Passthrough  SumFdbkVariant=Disabled  SumVariant=Sum_PID
  z_PID : simulink/Continuous/PID Controller  Controller=PID  Form=Parallel  TimeDomain=Discrete-time  SampleTime=5e-4  IntegratorMethod=Forward Euler  FilterMethod=Forward Euler  ControllerParametersSource=internal  P=0.007  I=0.005  D=0.003  UseFilter=on  N=100  TunerSelectOption=Transfer Function Based (PID Tuner App)  InitialConditionSource=internal  InitialConditionForIntegrator=0  InitialConditionForFilter=0  DifferentiatorICPrevScaledInput=0  ExternalReset=none  TrackingMode=off  Kt=1  LimitOutput=off  UpperSaturationLimit=inf  LowerSaturationLimit=-inf  LinearizeAsGain=on  AntiWindupMode=none  Kb=1  POutMin=[]  POutMax=[]  IOutMin=[]  IOutMax=[]  DOutMin=[]  DOutMax=[]  NOutMin=[]  NOutMax=[]  SumOutMin=[]  SumOutMax=[]  SaturationOutMin=[]  SaturationOutMax=[]  PParamMin=[]  PParamMax=[]  IParamMin=[]  IParamMax=[]  DParamMin=[]  DParamMax=[]  NParamMin=[]  NParamMax=[]  KbParamMin=[]  KbParamMax=[]  KtParamMin=[]  KtParamMax=[]  KbOutMin=[]  KbOutMax=[]  KtOutMin=[]  KtOutMax=[]  IntegratorOutMin=[]  IntegratorOutMax=[]  FilterOutMin=[]  FilterOutMax=[]  SumI1OutMin=[]  SumI1OutMax=[]  SumI2OutMin=[]  SumI2OutMax=[]  SumI3OutMin=[]  SumI3OutMax=[]  SumI4OutMin=[]  SumI4OutMax=[]  SumDOutMin=[]  SumDOutMax=[]  DifferentiatorOutMin=[]  DifferentiatorOutMax=[]  FilterDiffOutCoefMin=[]  FilterDiffOutCoefMax=[]  ReciprocalOutMin=[]  ReciprocalOutMax=[]  SumDenOutMin=[]  SumDenOutMax=[]  SumNumOutMin=[]  SumNumOutMax=[]  DivideOutMin=[]  DivideOutMax=[]  IntegratorContinuousStateAttributes=''  IntegratorStateMustResolveToSignalObject=off  IntegratorRTWStateStorageClass=Auto  FilterContinuousStateAttributes=''  FilterStateMustResolveToSignalObject=off  FilterRTWStateStorageClass=Auto  ParallelPVariant=InternalParameters  IdealPVariant=Disabled  IVariant=InternalParameters  DVariant=InternalParameters  IntegratorVariant=Discrete  SatVariant=Disabled  AWVariant=Passthrough  PCopyVariant=Disabled  TRVariant=Disabled  FdbkBlocksVariant=Forward  IdealPFdbkVariant=Disabled  SatFdbkVariant=Disabled  DerivativeFilterVariant=ForwardEulerFilter  NVariant=InternalParameters  NCopyVariant=Disabled  FilterICVariant=InternalICsFilter  IntegratorICVariant=InternalICs  ExternalResetVariant=Disabled  TRSumVariant=Passthrough  SumFdbkVariant=Disabled  SumVariant=Sum_PID
  omega1 : Outport
  omega2 : Outport  Port=2
  omega3 : Outport  Port=3
  omega4 : Outport  Port=4
  wires:
  Gain/1 -> Add3/1, Add2/1, Add1/1, Add/1
  Gain3/1 -> Add/3, Add1/3, Add3/3, Add2/3
  Gain2/1 -> Add3/2, Add2/2, Add/2, Add1/2
  Sum1/1 -> theta_PID/1
  Sum/1 -> alpha_PID/1
  Gain1/1 -> Add/4, Add1/4, Add2/4, Add3/4
  world to body - x/1(converted value) -> x_PID/1
  alpha_PID/1 -> Gain2/1
  theta_PID/1 -> Gain3/1
  phi_PID/1 -> Gain1/1
  world to body - z/1(converted value) -> z_PID/1
  y_PID/1 -> Sum/2
  x_PID/1 -> Sum1/2
  world to body - y/1(converted value) -> y_PID/1
  z_PID/1 -> Gain/1
  x_e/1 -> world to body - y/1(x_e), world to body - x/1(x_e), world to body - z/1(x_e)
  y_e/1 -> world to body - x/2(y_e), world to body - y/2(y_e), world to body - z/2(y_e)
  z_e/1 -> world to body - x/3(z_e), world to body - y/3(z_e), world to body - z/3(z_e)
  alpha/1 -> Sum/1, world to body - x/4(alpha), world to body - y/4(alpha), world to body - z/4(alpha)
  theta/1 -> Sum1/1, world to body - x/5(theta), world to body - y/5(theta), world to body - z/5(theta)
  phi/1 -> world to body - x/6(phi), world to body - y/6(phi), world to body - z/6(phi)
  phi_e/1 -> phi_PID/1
  Add/1 -> omega1/1
  Add1/1 -> omega2/1
  Add2/1 -> omega3/1
  Add3/1 -> omega4/1

== system Dron_pid_XY/Desired values/alpha_d (roll) ==
  Demux : Demux  Tag=STV Demux  Outputs=1
  FromWs : FromWorkspace  Tag=STV FromWs  VariableName=tuvar  SampleTime=0
      SigBuilderData=|
      | common.afterFinalStr = 'Extrapolate'
      | common.sampleTime = 0
      | dataSet.timeRange = [0 100]
      | dataSet.name = 'Group 1'
      | sbobj.Groups.Name = 'Group 1'
      | sbobj.Groups.Signals.Name = 'Signal 1'
      | sbobj.Groups.Signals.XData = [0 100]
      | sbobj.Groups.Signals.YData = [0 0]
      | sbobj.Groups.TimeRange = [0 100]
  Signal 1 : Outport  Tag=STV Outport
  wires:
  Demux/1 -> Signal 1/1
  FromWs/1 -> Demux/1

== system Dron_pid_XY/Desired values/phi_d (yaw) ==
  Demux : Demux  Tag=STV Demux  Outputs=1
  FromWs : FromWorkspace  Tag=STV FromWs  VariableName=tuvar  SampleTime=0
      SigBuilderData=|
      | common.afterFinalStr = 'Extrapolate'
      | common.sampleTime = 0
      | dataSet.timeRange = [0 100]
      | dataSet.name = 'Group 1'
      | sbobj.Groups.Name = 'Group 1'
      | sbobj.Groups.Signals.Name = 'Signal 1'
      | sbobj.Groups.Signals.XData = [0 100]
      | sbobj.Groups.Signals.YData = [0 0]
      | sbobj.Groups.TimeRange = [0 100]
  Signal 1 : Outport  Tag=STV Outport
  wires:
  Demux/1 -> Signal 1/1
  FromWs/1 -> Demux/1

== system Dron_pid_XY/Desired values/theta_d (pitch) ==
  Demux : Demux  Tag=STV Demux  Outputs=1
  FromWs : FromWorkspace  Tag=STV FromWs  VariableName=tuvar  SampleTime=0
      SigBuilderData=|
      | common.afterFinalStr = 'Extrapolate'
      | common.sampleTime = 0
      | dataSet.timeRange = [0 100]
      | dataSet.name = 'Group 1'
      | sbobj.Groups.Name = 'Group 1'
      | sbobj.Groups.Signals.Name = 'Signal 1'
      | sbobj.Groups.Signals.XData = [0 100]
      | sbobj.Groups.Signals.YData = [0 0]
      | sbobj.Groups.TimeRange = [0 100]
  Signal 1 : Outport  Tag=STV Outport
  wires:
  Demux/1 -> Signal 1/1
  FromWs/1 -> Demux/1

== system Dron_pid_XY/Desired values/x_d position ==
  Demux : Demux  Tag=STV Demux  Outputs=1
  FromWs : FromWorkspace  Tag=STV FromWs  VariableName=tuvar  SampleTime=0
      SigBuilderData=|
      | common.afterFinalStr = 'Extrapolate'
      | common.sampleTime = 0
      | dataSet.timeRange = [0 100]
      | dataSet.name = 'Group 1'
      | sbobj.Groups.Name = 'Group 1'
      | sbobj.Groups.Signals.Name = 'Signal 1'
      | sbobj.Groups.Signals.XData = [0 15 20 25 30 35 40 45 50 55 100]
      | sbobj.Groups.Signals.YData = [0 0 2 4 6 6 4 2 0 0 0]
      | sbobj.Groups.TimeRange = [0 100]
  Signal 1 : Outport  Tag=STV Outport
  wires:
  Demux/1 -> Signal 1/1
  FromWs/1 -> Demux/1

== system Dron_pid_XY/Desired values/y_d position ==
  Demux : Demux  Tag=STV Demux  Outputs=1
  FromWs : FromWorkspace  Tag=STV FromWs  VariableName=tuvar  SampleTime=0
      SigBuilderData=|
      | common.afterFinalStr = 'Extrapolate'
      | common.sampleTime = 0
      | dataSet.timeRange = [0 100]
      | dataSet.name = 'Group 1'
      | sbobj.Groups.Name = 'Group 1'
      | sbobj.Groups.Signals.Name = 'Signal 1'
      | sbobj.Groups.Signals.XData = [0 15 20 25 30 35 40 45 50 100]
      | sbobj.Groups.Signals.YData = [0 0 2 2 0 -2 -4 -4 -2 -2]
      | sbobj.Groups.TimeRange = [0 100]
  Signal 1 : Outport  Tag=STV Outport
  wires:
  Demux/1 -> Signal 1/1
  FromWs/1 -> Demux/1

== system Dron_pid_XY/Desired values/z_d position ==
  Demux : Demux  Tag=STV Demux  Outputs=1
  FromWs : FromWorkspace  Tag=STV FromWs  VariableName=tuvar  SampleTime=0
      SigBuilderData=|
      | common.afterFinalStr = 'Extrapolate'
      | common.sampleTime = 0
      | dataSet.timeRange = [0 100]
      | dataSet.name = 'Group 1'
      | sbobj.Groups.Name = 'Group 1'
      | sbobj.Groups.Signals.Name = 'Signal 1'
      | sbobj.Groups.Signals.XData = [0 10 85 95 100]
      | sbobj.Groups.Signals.YData = [0 5 5 0 0]
      | sbobj.Groups.TimeRange = [0 100]
  Signal 1 : Outport  Tag=STV Outport
  wires:
  Demux/1 -> Signal 1/1
  FromWs/1 -> Demux/1

== system Dron_pid_XY/Linear accelerations/Body to world - x ==
  alpha : Inport
  theta : Inport  Port=2
  "phi " : Inport  Port=3
  X body acceleration : Inport  Port=4
  Add1 : Sum
  Cos4 : Trigonometry  Operator=cos
  Cos5 : Trigonometry  Operator=cos
  Product : Product
  Product1 : Product  Inputs=3
  Product4 : Product
  Sin3 : Trigonometry
  Sin4 : Trigonometry
  Sin5 : Trigonometry
  converted value : Outport
  wires:
  Cos4/1 -> Product1/2
  Sin5/1 -> Product4/1
  theta/1 -> Sin3/1
  Product4/1 -> Add1/1
  Cos5/1 -> Product1/1
  "phi "/1 -> Cos4/1, Sin4/1
  alpha/1 -> Cos5/1, Sin5/1
  Sin4/1 -> Product4/2
  Product1/1 -> Add1/2
  Sin3/1 -> Product1/3
  Add1/1 -> Product/1
  Product/1 -> converted value/1
  X body acceleration/1 -> Product/2

== system Dron_pid_XY/Linear accelerations/Body to world - y ==
  alpha : Inport
  theta : Inport  Port=2
  phi : Inport  Port=3
  Y body acceleration : Inport  Port=4
  Add2 : Sum
  Cos : Trigonometry  Operator=cos
  Cos3 : Trigonometry  Operator=cos
  Product : Product
  Product2 : Product  Inputs=3
  Product5 : Product
  Sin : Trigonometry
  Sin1 : Trigonometry
  Sin2 : Trigonometry
  converted value : Outport
  wires:
  Sin2/1 -> Product5/1
  Sin/1 -> Product2/3
  Product5/1 -> Add2/1
  theta/1 -> Sin/1
  Sin1/1 -> Product2/2
  Cos3/1 -> Product2/1
  phi/1 -> Cos/1, Sin1/1
  Product2/1 -> Add2/2
  Add2/1 -> Product/1
  alpha/1 -> Cos3/1, Sin2/1
  Product/1 -> converted value/1
  Y body acceleration/1 -> Product/2
  Cos/1 -> Product5/2

== system Dron_pid_XY/Linear accelerations/Body to world - z ==
  alpha : Inport
  theta : Inport  Port=2
  Z body acceleration : Inport  Port=3
  Cos : Trigonometry  Operator=cos
  Cos1 : Trigonometry  Operator=cos
  Product : Product  Inputs=3
  converted value : Outport
  wires:
  theta/1 -> Cos/1
  alpha/1 -> Cos1/1
  Cos1/1 -> Product/2
  Cos/1 -> Product/1
  Product/1 -> converted value/1
  Z body acceleration/1 -> Product/3

== system Dron_pid_XY/Linear and angular errors/X regulation quality indicators ==
  x_e : Inport
  Abs : Abs
  Integrator : Integrator
  Integrator1 : Integrator
  Square : Math  Operator=square  SaturateOnIntegerOverflow=on
  To Workspace : ToWorkspace  VariableName=x_ise  SampleTime=-1
  To Workspace1 : ToWorkspace  VariableName=x_iae  SampleTime=-1
  wires:
  Integrator/1 -> To Workspace/1
  x_e/1 -> Square/1, Abs/1
  Square/1 -> Integrator/1
  Integrator1/1 -> To Workspace1/1
  Abs/1 -> Integrator1/1

== system Dron_pid_XY/Linear and angular errors/Y regulation quality indicators ==
  y_e : Inport
  Abs : Abs
  Integrator : Integrator
  Integrator1 : Integrator
  Square : Math  Operator=square  SaturateOnIntegerOverflow=on
  To Workspace : ToWorkspace  VariableName=y_ise  SampleTime=-1
  To Workspace1 : ToWorkspace  VariableName=y_iae  SampleTime=-1
  wires:
  Abs/1 -> Integrator1/1
  Integrator1/1 -> To Workspace1/1
  Square/1 -> Integrator/1
  y_e/1 -> Abs/1, Square/1
  Integrator/1 -> To Workspace/1

== system Dron_pid_XY/Linear and angular errors/Z regulation quality indicators ==
  z_e : Inport
  Abs : Abs
  Integrator : Integrator
  Integrator1 : Integrator
  Square : Math  Operator=square  SaturateOnIntegerOverflow=on
  To Workspace : ToWorkspace  VariableName=z_ise  SampleTime=-1
  To Workspace1 : ToWorkspace  VariableName=z_iae  SampleTime=-1
  wires:
  Integrator/1 -> To Workspace/1
  z_e/1 -> Square/1, Abs/1
  Square/1 -> Integrator/1
  Integrator1/1 -> To Workspace1/1
  Abs/1 -> Integrator1/1

== system Dron_pid_XY/Motors Control/Torque disturbance ==
  Disturbance gain : Gain
  Disturbance inertia : TransferFcn  Denominator=[3 3 1]
  Disturbance model : powerlib_extras/Control  Blocks/Timer  t=[0 0.1 10 30 45 55 65 70 75 85 95]  e=[0 0.01 0.05 0.1 0.2 0.1 0.05 0.02 0.05 0.1 0.05]
      settings: SourceProductName=Simscape Electrical  SourceProductBaseCode=PS
  Disturbance plot : Scope
  Product : Product
  Random signal : UniformRandomNumber  Minimum=0.8  Maximum=1.2  Seed=233839  SampleTime=2
  To workspace : ToWorkspace  VariableName=disturbance  SampleTime=1e-4
  Zero-Order Hold2 : ZeroOrderHold  SampleTime=1e-4
  Sig_out : Outport
  wires:
  Random signal/1 -> Product/2
  Product/1 -> Disturbance inertia/1
  Disturbance model/1 -> Product/1
  Zero-Order Hold2/1 -> Disturbance gain/1
  Disturbance gain/1 -> To workspace/1, Disturbance plot/1, Sig_out/1
  Disturbance inertia/1 -> Zero-Order Hold2/1

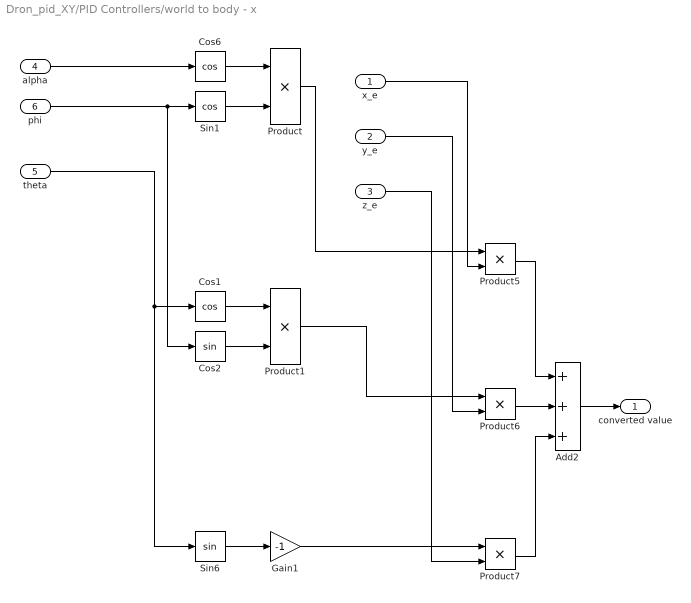
== system Dron_pid_XY/PID Controllers/world to body - x ==
  x_e : Inport
  y_e : Inport  Port=2
  z_e : Inport  Port=3
  alpha : Inport  Port=4
  theta : Inport  Port=5
  phi : Inport  Port=6
  Add2 : Sum  Inputs=+++
  Cos1 : Trigonometry  Operator=cos
  Cos2 : Trigonometry
  Cos6 : Trigonometry  Operator=cos
  Gain1 : Gain  Gain=-1
  Product{,1,5..7} (5 alike) : Product
  Sin1 : Trigonometry  Operator=cos
  Sin6 : Trigonometry
  converted value : Outport
  wires:
  Cos1/1 -> Product1/1
  x_e/1 -> Product5/2
  Add2/1 -> converted value/1
  Product5/1 -> Add2/1
  Sin1/1 -> Product/2
  Product6/1 -> Add2/2
  Cos6/1 -> Product/1
  z_e/1 -> Product7/2
  y_e/1 -> Product6/2
  Product7/1 -> Add2/3
  phi/1 -> Cos2/1, Sin1/1
  Cos2/1 -> Product1/2
  Sin6/1 -> Gain1/1
  theta/1 -> Cos1/1, Sin6/1
  Product/1 -> Product5/1
  Gain1/1 -> Product7/1
  Product1/1 -> Product6/1
  alpha/1 -> Cos6/1

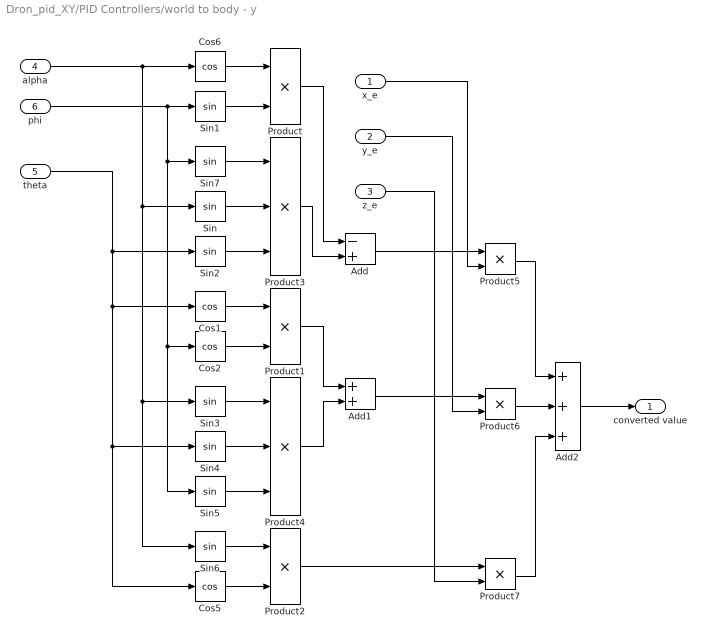
== system Dron_pid_XY/PID Controllers/world to body - y ==
  x_e : Inport
  y_e : Inport  Port=2
  z_e : Inport  Port=3
  alpha : Inport  Port=4
  theta : Inport  Port=5
  phi : Inport  Port=6
  Add : Sum  Inputs=-+
  Add1 : Sum
  Add2 : Sum  Inputs=+++
  Cos{1..2,5..6} (4 alike) : Trigonometry  Operator=cos
  Product{,1..2,5..7} (6 alike) : Product
  Product3 : Product  Inputs=3
  Product4 : Product  Inputs=3
  Sin{,1..7} (8 alike) : Trigonometry
  converted value : Outport
  wires:
  phi/1 -> Sin7/1, Sin5/1, Cos2/1, Sin1/1
  Cos1/1 -> Product1/1
  Sin7/1 -> Product3/1
  Sin6/1 -> Product2/1
  alpha/1 -> Cos6/1, Sin/1, Sin6/1, Sin3/1
  Cos6/1 -> Product/1
  z_e/1 -> Product7/2
  Sin/1 -> Product3/2
  Cos5/1 -> Product2/2
  Product4/1 -> Add1/2
  Product6/1 -> Add2/2
  Product1/1 -> Add1/1
  Sin5/1 -> Product4/3
  Sin1/1 -> Product/2
  Sin2/1 -> Product3/3
  Product7/1 -> Add2/3
  Add/1 -> Product5/1
  Product/1 -> Add/1
  Product2/1 -> Product7/1
  Cos2/1 -> Product1/2
  Add1/1 -> Product6/1
  x_e/1 -> Product5/2
  Sin4/1 -> Product4/2
  Product3/1 -> Add/2
  theta/1 -> Cos1/1, Cos5/1, Sin4/1, Sin2/1
  Sin3/1 -> Product4/1
  y_e/1 -> Product6/2
  Product5/1 -> Add2/1
  Add2/1 -> converted value/1

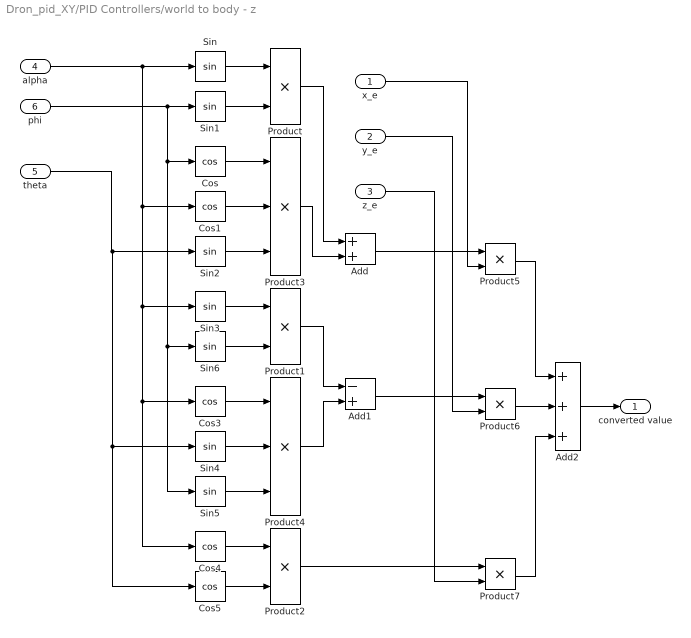
== system Dron_pid_XY/PID Controllers/world to body - z ==
  x_e : Inport
  y_e : Inport  Port=2
  z_e : Inport  Port=3
  alpha : Inport  Port=4
  theta : Inport  Port=5
  phi : Inport  Port=6
  Add : Sum
  Add1 : Sum  Inputs=-+
  Add2 : Sum  Inputs=+++
  Cos{,1,3..5} (5 alike) : Trigonometry  Operator=cos
  Product{,1..2,5..7} (6 alike) : Product
  Product3 : Product  Inputs=3
  Product4 : Product  Inputs=3
  Sin{,1..6} (7 alike) : Trigonometry
  converted value : Outport
  wires:
  Product1/1 -> Add1/1
  Product/1 -> Add/1
  Add/1 -> Product5/1
  Add1/1 -> Product6/1
  Product2/1 -> Product7/1
  Add2/1 -> converted value/1
  Product7/1 -> Add2/3
  Product6/1 -> Add2/2
  Product5/1 -> Add2/1
  Sin/1 -> Product/1
  alpha/1 -> Sin/1, Cos4/1, Cos3/1, Sin3/1, Cos1/1
  Sin1/1 -> Product/2
  Cos/1 -> Product3/1
  Cos1/1 -> Product3/2
  Sin2/1 -> Product3/3
  theta/1 -> Cos5/1, Sin4/1, Sin2/1
  Product3/1 -> Add/2
  Product4/1 -> Add1/2
  Sin3/1 -> Product1/1
  Sin6/1 -> Product1/2
  Cos3/1 -> Product4/1
  Sin4/1 -> Product4/2
  Sin5/1 -> Product4/3
  phi/1 -> Sin6/1, Sin5/1, Cos/1, Sin1/1
  Cos4/1 -> Product2/1
  Cos5/1 -> Product2/2
  x_e/1 -> Product5/2
  y_e/1 -> Product6/2
  z_e/1 -> Product7/2
